simulink model "SomanetTuning"  (R2016b)
settings: Solver=FixedStepDiscrete  StartTime=0.0  StopTime=inf  FixedStep=0.002  RelTol=1e-3  EnableMultiTasking=on
libraries: slrtlib x14, dspstat3 x2, xpcethercatlib x1
(part 1 of 2)
settings Model: SimulationMode=external  Creator=march  LastModifiedBy=march
settings SolverCC: EnableConcurrentExecution=on  AutoInsertRateTranBlk=on
settings DataIOCC: SaveFormat=StructureWithTime
settings OptimizationCC: BlockReduction=off  OptimizeBlockIOStorage=off  BufferReuse=off  GlobalBufferReuse=off  ExpressionFolding=off  LocalBlockOutputs=off
settings HardwareCC: ProdBitPerPointer=32  ProdBitPerSizeT=32  ProdBitPerPtrDiffT=32  ProdLargestAtomicFloat=None  ProdWordSize=32  ProdLongLongMode=on  ProdHWDeviceType=Generic->32-bit x86 compatible
settings RTWCC: SystemTargetFile=slrt.tlc  TemplateMakefile=slrt_default_tmf  PostCodeGenCommand=SomanetTuning_make_rtw_hook  Description=Simulink Real-Time  RTWVerbose=off  CodeExecutionProfiling=on  RTWCompilerOptimization=on
settings SimulinkRealTimeCC: xPCModelTimeoutSecs=20

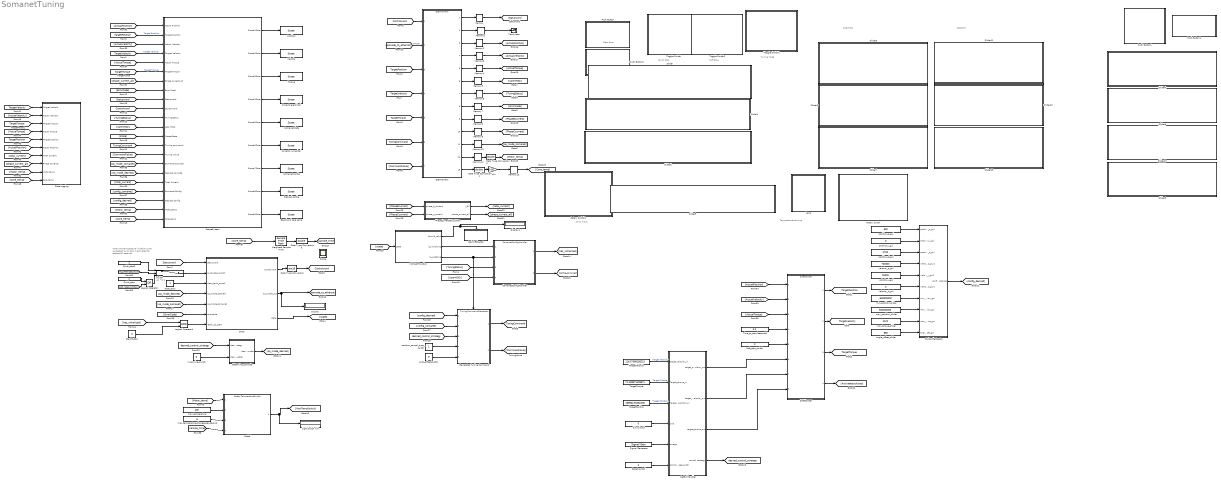
== system SomanetTuning ==
  note: VELOCITY
  note: POSITION
  note: Sinus Input
  note: Tuning Mode
  note: Quick Stop
  note: Clear Error
  note: When the temperature limitations are exceeded quick stop is activated for atleast 60 seconds
  note: Temperature-warning
  note: Soft Stop
  Board and core temp : slrtlib/Displays and Logging/Scope   scopeno=9  scopetype=Target  autostart=on  viewmode=Graphical rolling  formatstr='%15.6f'  grid=on  ylimits=[20,100]  nosamples=250  noprepostsamples=0  interleave=1  triggermode=FreeRun  triggersignal=1  trigsignalfromport=off  triggerlevel=0.0  triggerslope=Either  triggerscope=1  triggersample=0  filename=data.dat  mode=Lazy  writesize=512  autorestart=off  dynamicfilemode=off  maxwritefilesize=512*1024^2
  Chart : Stateflow chart  TreatAsAtomicUnit=on
  Currents graphical : slrtlib/Displays and Logging/Scope   scopeno=4  scopetype=Target  autostart=on  viewmode=Graphical sliding  formatstr='%15.6f'  grid=on  ylimits=[-30000,30000]  nosamples=500  noprepostsamples=0  interleave=1  triggermode=FreeRun  triggersignal=1  trigsignalfromport=off  triggerlevel=0.0  triggerslope=Either  triggerscope=1  triggersample=0  filename=data.dat  mode=Lazy  writesize=512  autorestart=off  dynamicfilemode=off  maxwritefilesize=512*1024^2
  Currents numerical : slrtlib/Displays and Logging/Scope   scopeno=6  scopetype=Target  autostart=on  viewmode=Numerical  formatstr='%15.6f'  grid=on  ylimits=[0,15000]  nosamples=500  noprepostsamples=0  interleave=1  triggermode=FreeRun  triggersignal=1  trigsignalfromport=off  triggerlevel=0.0  triggerslope=Either  triggerscope=1  triggersample=0  filename=data.dat  mode=Lazy  writesize=512  autorestart=off  dynamicfilemode=off  maxwritefilesize=512*1024^2
  Data Type Conversion : DataTypeConversion  OutDataTypeStr=uint16
  Data Type Conversion1 : DataTypeConversion  OutDataTypeStr=double
  Data Type Conversion2 : DataTypeConversion  OutDataTypeStr=double
  Data Type Conversion3 : DataTypeConversion  OutDataTypeStr=double
  Data logging : Subsystem
  Desired config : slrtlib/Displays and Logging/Scope   scopeno=8  scopetype=Target  autostart=on  viewmode=Numerical  formatstr='%15.0f'  grid=on  ylimits=[-600,600]  nosamples=500  noprepostsamples=0  interleave=1  triggermode=FreeRun  triggersignal=1  trigsignalfromport=off  triggerlevel=0.0  triggerslope=Either  triggerscope=1  triggersample=0  filename=data.dat  mode=Lazy  writesize=512  autorestart=off  dynamicfilemode=off  maxwritefilesize=512*1024^2
  Display : Display
  Display1 : Display
  EcatHandler : ModelReference  ModelNameDialog=EcatHandler  SimulationMode=Normal  ModelReferenceVersion=1.312
  Gain : Gain  Gain=0.05
  Generates Tuning Command : ModelReference  ModelNameDialog=TuningCommandGenerator.slx  SimulationMode=Normal  ModelReferenceVersion=1.298  EnablePortName=Enable  EnablePortStatesWhenEnabling=held
  GuiConfigCreator : Subsystem  TreatAsAtomicUnit=on
  Lamp : Subsystem  DialogController=hmiCreateDDGDialog  IsWebBlock=on  mask(MWDashboardBlock){webBlockId=994b938f-f4a1-444b-8998-3c3fe0212c8b, webBlockType=lamp, ShowInLibBrowser=on, ShowInitialText=on, HMISrcModelName=SomanetTuning}
      mask prompts: webBlockType "WebBlock Type"; HMISrcModelName "Source Model"
      mask help: SimulinkHMI:dialogs:LampDialogDesc
      mask Help: helpview([docroot '/mapfiles/simulink.map'], 'hmi_lamp')
      mask Display:
      | if strcmp(get_param(bdroot(gcb),'BlockDiagramType'), 'library')
      |     image([(matlabroot) '/toolbox/simulink/hmi/icons/Lamp.png']);
      | end
  Light Switch link : Display
  Logical Operator : Logic  Operator=OR  AllPortsSameDT=off  OutDataTypeStr=boolean
  Logical Operator1 : Logic  AllPortsSameDT=off  OutDataTypeStr=boolean
  MATLAB Function : MATLAB Function  TreatAsAtomicUnit=on
  Memory{,1..12} (13 alike) : Memory
  Model : ModelReference  ModelNameDialog=SafetyTemperatureSwitch.slx  SimulationMode=Normal  ModelReferenceVersion=1.310
  PhaseCurrentCalculation : Subsystem
  Position : slrtlib/Displays and Logging/Scope   scopeno=1  scopetype=Target  autostart=on  viewmode=Graphical sliding  formatstr='%15.6f'  grid=on  ylimits=[-5e6,5e6]  nosamples=500  noprepostsamples=0  interleave=1  triggermode=FreeRun  triggersignal=1  trigsignalfromport=off  triggerlevel=0.0  triggerslope=Either  triggerscope=1  triggersample=0  filename=data.dat  mode=Lazy  writesize=512  autorestart=off  dynamicfilemode=off  maxwritefilesize=512*1024^2
  Push Button : Subsystem  DialogController=hmiCreateDDGDialog  IsWebBlock=on  mask(MWDashboardBlock){webBlockId=356734de-af8c-46d0-90c2-8e8f664c98d9, webBlockType=pushbutton, ShowInLibBrwoser=on, ShowInitialText=on, HMISrcModelName=SomanetTuning}
      mask prompts: webBlockId "WebBlock Id"; webBlockType "WebBlock Type"; HMISrcModelName "Source Model"
      mask help: SimulinkHMI:dialogs:PushButtonDialogDesc
      mask Help: helpview([docroot '/mapfiles/simulink.map'], 'hmi_push_button')
      mask Display:
      | model = bdroot(gcb);
      | if strcmp(get_param(model,'BlockDiagramType'), 'library')
      |     image([(matlabroot) '/toolbox/simulink/hmi/icons/PushButton.png']);
      | end
  Push Button1 : Subsystem  DialogController=hmiCreateDDGDialog  IsWebBlock=on  mask(MWDashboardBlock){webBlockId=183612d4-71ac-4f8a-91dd-632476c1d2bb, webBlockType=pushbutton, ShowInLibBrwoser=on, ShowInitialText=on, HMISrcModelName=SomanetTuning}
      mask prompts: webBlockId "WebBlock Id"; webBlockType "WebBlock Type"; HMISrcModelName "Source Model"
      mask help: SimulinkHMI:dialogs:PushButtonDialogDesc
      mask Help: helpview([docroot '/mapfiles/simulink.map'], 'hmi_push_button')
      mask Display:
      | model = bdroot(gcb);
      | if strcmp(get_param(model,'BlockDiagramType'), 'library')
      |     image([(matlabroot) '/toolbox/simulink/hmi/icons/PushButton.png']);
      | end
  Push Button2 : Subsystem  DialogController=hmiCreateDDGDialog  IsWebBlock=on  mask(MWDashboardBlock){webBlockId=3a1387a3-9f18-4c83-b61d-eeb4a0f66ee7, webBlockType=pushbutton, ShowInLibBrwoser=on, ShowInitialText=on, HMISrcModelName=SomanetTuning}
      mask prompts: webBlockId "WebBlock Id"; webBlockType "WebBlock Type"; HMISrcModelName "Source Model"
      mask help: SimulinkHMI:dialogs:PushButtonDialogDesc
      mask Help: helpview([docroot '/mapfiles/simulink.map'], 'hmi_push_button')
      mask Display:
      | model = bdroot(gcb);
      | if strcmp(get_param(model,'BlockDiagramType'), 'library')
      |     image([(matlabroot) '/toolbox/simulink/hmi/icons/PushButton.png']);
      | end
  Push Button3 : Subsystem  DialogController=hmiCreateDDGDialog  IsWebBlock=on  mask(MWDashboardBlock){webBlockId=e281f3a8-d07c-4ea7-a33e-ce327e187917, webBlockType=pushbutton, ShowInLibBrwoser=on, ShowInitialText=on, HMISrcModelName=SomanetTuning}
      mask prompts: webBlockId "WebBlock Id"; webBlockType "WebBlock Type"; HMISrcModelName "Source Model"
      mask help: SimulinkHMI:dialogs:PushButtonDialogDesc
      mask Help: helpview([docroot '/mapfiles/simulink.map'], 'hmi_push_button')
      mask Display:
      | model = bdroot(gcb);
      | if strcmp(get_param(model,'BlockDiagramType'), 'library')
      |     image([(matlabroot) '/toolbox/simulink/hmi/icons/PushButton.png']);
      | end
  Quick_stop : Constant  OutDataTypeStr=boolean
  Quick_stop2 : Constant  OutDataTypeStr=boolean
  Reinit Ethercat : Subsystem
  Reset control : Constant  Value=0  OutDataTypeStr=int32
  Rotary Switch : Subsystem  DialogController=hmiCreateDDGDialog  IsWebBlock=on  mask(MWDashboardBlock){webBlockId=fa8f8082-b632-4cd3-875a-301596b55e06, webBlockType=discreteknob, ShowInLibBrowser=on, ShowInitialText=on, HMISrcModelName=SomanetTuning}
      mask prompts: webBlockId "WebBlock Id"; webBlockType "WebBlock Type"; HMISrcModelName "Source Model"
      mask help: SimulinkHMI:dialogs:DiscreteKnobDialogDesc
      mask Help: helpview([docroot '/mapfiles/simulink.map'], 'hmi_rotary_switch')
      mask Display:
      | model = bdroot(gcb);
      | if strcmp(get_param(model,'BlockDiagramType'), 'library')
      |     image([(matlabroot) '/toolbox/simulink/hmi/icons/DiscreteKnob.png']);
      | end
  Rotary Switch1 : Subsystem  DialogController=hmiCreateDDGDialog  IsWebBlock=on  mask(MWDashboardBlock){webBlockId=1d56b400-0412-44c3-8462-8cb9db8b7e4d, webBlockType=discreteknob, ShowInLibBrowser=on, ShowInitialText=on, HMISrcModelName=SomanetTuning}
      mask prompts: webBlockId "WebBlock Id"; webBlockType "WebBlock Type"; HMISrcModelName "Source Model"
      mask help: SimulinkHMI:dialogs:DiscreteKnobDialogDesc
      mask Help: helpview([docroot '/mapfiles/simulink.map'], 'hmi_rotary_switch')
      mask Display:
      | model = bdroot(gcb);
      | if strcmp(get_param(model,'BlockDiagramType'), 'library')
      |     image([(matlabroot) '/toolbox/simulink/hmi/icons/DiscreteKnob.png']);
      | end
  ScopeSystem : Subsystem
  SetGuiHandler : Subsystem
  Signal Generator : SignalGenerator  Frequency=0.281954887218
  "Sinus Input " : Constant  Value=0
  Slider : Subsystem  DialogController=hmiCreateDDGDialog  IsWebBlock=on  mask(MWDashboardBlock){webBlockId=d1263451-46af-4c55-8eeb-b2a1185fc98c, webBlockType=slider, ShowInLibBrowser=on, ShowInitialText=on, HMISrcModelName=SomanetTuning}
      mask prompts: webBlockId "WebBlock Id"; webBlockType "WebBlock Type"; HMISrcModelName "Source Model"
      mask help: SimulinkHMI:dialogs:SliderDialogDesc
      mask Help: helpview([docroot '/mapfiles/simulink.map'], 'hmi_slider')
      mask Display:
      | if strcmp(get_param(bdroot(gcb),'BlockDiagramType'), 'library')
      |     image([(matlabroot) '/toolbox/simulink/hmi/icons/Slider.png']);
      | end
  Slider1 : Subsystem  DialogController=hmiCreateDDGDialog  IsWebBlock=on  mask(MWDashboardBlock){webBlockId=e2636b5b-382c-42e0-acf3-b39c3266f57b, webBlockType=slider, ShowInLibBrowser=on, ShowInitialText=on, HMISrcModelName=SomanetTuning}
      mask prompts: webBlockId "WebBlock Id"; webBlockType "WebBlock Type"; HMISrcModelName "Source Model"
      mask help: SimulinkHMI:dialogs:SliderDialogDesc
      mask Help: helpview([docroot '/mapfiles/simulink.map'], 'hmi_slider')
      mask Display:
      | if strcmp(get_param(bdroot(gcb),'BlockDiagramType'), 'library')
      |     image([(matlabroot) '/toolbox/simulink/hmi/icons/Slider.png']);
      | end
  Slider10 : Subsystem  DialogController=hmiCreateDDGDialog  IsWebBlock=on  mask(MWDashboardBlock){webBlockId=def7d2a7-1287-4d64-81c3-00dc42338eac, webBlockType=slider, ShowInLibBrowser=on, ShowInitialText=on, HMISrcModelName=SomanetTuning}
      mask prompts: webBlockId "WebBlock Id"; webBlockType "WebBlock Type"; HMISrcModelName "Source Model"
      mask help: SimulinkHMI:dialogs:SliderDialogDesc
      mask Help: helpview([docroot '/mapfiles/simulink.map'], 'hmi_slider')
      mask Display:
      | if strcmp(get_param(bdroot(gcb),'BlockDiagramType'), 'library')
      |     image([(matlabroot) '/toolbox/simulink/hmi/icons/Slider.png']);
      | end
  Slider11 : Subsystem  DialogController=hmiCreateDDGDialog  IsWebBlock=on  mask(MWDashboardBlock){webBlockId=dc2b2cfc-71ae-4ea0-a0f2-7e0884df10cf, webBlockType=slider, ShowInLibBrowser=on, ShowInitialText=on, HMISrcModelName=SomanetTuning}
      mask prompts: webBlockId "WebBlock Id"; webBlockType "WebBlock Type"; HMISrcModelName "Source Model"
      mask help: SimulinkHMI:dialogs:SliderDialogDesc
      mask Help: helpview([docroot '/mapfiles/simulink.map'], 'hmi_slider')
      mask Display:
      | if strcmp(get_param(bdroot(gcb),'BlockDiagramType'), 'library')
      |     image([(matlabroot) '/toolbox/simulink/hmi/icons/Slider.png']);
      | end
  Slider12 : Subsystem  DialogController=hmiCreateDDGDialog  IsWebBlock=on  mask(MWDashboardBlock){webBlockId=7ae4c4dc-b42e-45e0-b891-75a3f1e5fd6f, webBlockType=slider, ShowInLibBrowser=on, ShowInitialText=on, HMISrcModelName=SomanetTuning}
      mask prompts: webBlockId "WebBlock Id"; webBlockType "WebBlock Type"; HMISrcModelName "Source Model"
      mask help: SimulinkHMI:dialogs:SliderDialogDesc
      mask Help: helpview([docroot '/mapfiles/simulink.map'], 'hmi_slider')
      mask Display:
      | if strcmp(get_param(bdroot(gcb),'BlockDiagramType'), 'library')
      |     image([(matlabroot) '/toolbox/simulink/hmi/icons/Slider.png']);
      | end
  Slider13 : Subsystem  DialogController=hmiCreateDDGDialog  IsWebBlock=on  mask(MWDashboardBlock){webBlockId=f6d04e87-2e98-45c4-b429-031f5ea3085d, webBlockType=slider, ShowInLibBrowser=on, ShowInitialText=on, HMISrcModelName=SomanetTuning}
      mask prompts: webBlockId "WebBlock Id"; webBlockType "WebBlock Type"; HMISrcModelName "Source Model"
      mask help: SimulinkHMI:dialogs:SliderDialogDesc
      mask Help: helpview([docroot '/mapfiles/simulink.map'], 'hmi_slider')
      mask Display:
      | if strcmp(get_param(bdroot(gcb),'BlockDiagramType'), 'library')
      |     image([(matlabroot) '/toolbox/simulink/hmi/icons/Slider.png']);
      | end
  Slider2 : Subsystem  DialogController=hmiCreateDDGDialog  IsWebBlock=on  mask(MWDashboardBlock){webBlockId=71234142-cef9-4b37-b6ab-ce5d7e36af05, webBlockType=slider, ShowInLibBrowser=on, ShowInitialText=on, HMISrcModelName=SomanetTuning}
      mask prompts: webBlockId "WebBlock Id"; webBlockType "WebBlock Type"; HMISrcModelName "Source Model"
      mask help: SimulinkHMI:dialogs:SliderDialogDesc
      mask Help: helpview([docroot '/mapfiles/simulink.map'], 'hmi_slider')
      mask Display:
      | if strcmp(get_param(bdroot(gcb),'BlockDiagramType'), 'library')
      |     image([(matlabroot) '/toolbox/simulink/hmi/icons/Slider.png']);
      | end
  Slider3 : Subsystem  DialogController=hmiCreateDDGDialog  IsWebBlock=on  mask(MWDashboardBlock){webBlockId=9cddd46d-1cb7-4126-ab3d-ebd7afdeb18b, webBlockType=slider, ShowInLibBrowser=on, ShowInitialText=on, HMISrcModelName=SomanetTuning}
      mask prompts: webBlockId "WebBlock Id"; webBlockType "WebBlock Type"; HMISrcModelName "Source Model"
      mask help: SimulinkHMI:dialogs:SliderDialogDesc
      mask Help: helpview([docroot '/mapfiles/simulink.map'], 'hmi_slider')
      mask Display:
      | if strcmp(get_param(bdroot(gcb),'BlockDiagramType'), 'library')
      |     image([(matlabroot) '/toolbox/simulink/hmi/icons/Slider.png']);
      | end
  Slider4 : Subsystem  DialogController=hmiCreateDDGDialog  IsWebBlock=on  mask(MWDashboardBlock){webBlockId=fa1a1418-0503-4b20-b29d-6741a8e61eb2, webBlockType=slider, ShowInLibBrowser=on, ShowInitialText=on, HMISrcModelName=SomanetTuning}
      mask prompts: webBlockId "WebBlock Id"; webBlockType "WebBlock Type"; HMISrcModelName "Source Model"
      mask help: SimulinkHMI:dialogs:SliderDialogDesc
      mask Help: helpview([docroot '/mapfiles/simulink.map'], 'hmi_slider')
      mask Display:
      | if strcmp(get_param(bdroot(gcb),'BlockDiagramType'), 'library')
      |     image([(matlabroot) '/toolbox/simulink/hmi/icons/Slider.png']);
      | end
  Slider5 : Subsystem  DialogController=hmiCreateDDGDialog  IsWebBlock=on  mask(MWDashboardBlock){webBlockId=e24694ff-6856-4d6d-8c39-63b50901b388, webBlockType=slider, ShowInLibBrowser=on, ShowInitialText=on, HMISrcModelName=SomanetTuning}
      mask prompts: webBlockId "WebBlock Id"; webBlockType "WebBlock Type"; HMISrcModelName "Source Model"
      mask help: SimulinkHMI:dialogs:SliderDialogDesc
      mask Help: helpview([docroot '/mapfiles/simulink.map'], 'hmi_slider')
      mask Display:
      | if strcmp(get_param(bdroot(gcb),'BlockDiagramType'), 'library')
      |     image([(matlabroot) '/toolbox/simulink/hmi/icons/Slider.png']);
      | end
  Slider6 : Subsystem  DialogController=hmiCreateDDGDialog  IsWebBlock=on  mask(MWDashboardBlock){webBlockId=8e804c44-8f02-4255-850c-29e295587076, webBlockType=slider, ShowInLibBrowser=on, ShowInitialText=on, HMISrcModelName=SomanetTuning}
      mask prompts: webBlockId "WebBlock Id"; webBlockType "WebBlock Type"; HMISrcModelName "Source Model"
      mask help: SimulinkHMI:dialogs:SliderDialogDesc
      mask Help: helpview([docroot '/mapfiles/simulink.map'], 'hmi_slider')
      mask Display:
      | if strcmp(get_param(bdroot(gcb),'BlockDiagramType'), 'library')
      |     image([(matlabroot) '/toolbox/simulink/hmi/icons/Slider.png']);
      | end
  Slider7 : Subsystem  DialogController=hmiCreateDDGDialog  IsWebBlock=on  mask(MWDashboardBlock){webBlockId=44154478-d107-4041-943a-7a09b0b07a14, webBlockType=slider, ShowInLibBrowser=on, ShowInitialText=on, HMISrcModelName=SomanetTuning}
      mask prompts: webBlockId "WebBlock Id"; webBlockType "WebBlock Type"; HMISrcModelName "Source Model"
      mask help: SimulinkHMI:dialogs:SliderDialogDesc
      mask Help: helpview([docroot '/mapfiles/simulink.map'], 'hmi_slider')
      mask Display:
      | if strcmp(get_param(bdroot(gcb),'BlockDiagramType'), 'library')
      |     image([(matlabroot) '/toolbox/simulink/hmi/icons/Slider.png']);
      | end
  Slider8 : Subsystem  DialogController=hmiCreateDDGDialog  IsWebBlock=on  mask(MWDashboardBlock){webBlockId=b2209b26-3c3d-4464-9b10-a7343f526e76, webBlockType=slider, ShowInLibBrowser=on, ShowInitialText=on, HMISrcModelName=SomanetTuning}
      mask prompts: webBlockId "WebBlock Id"; webBlockType "WebBlock Type"; HMISrcModelName "Source Model"
      mask help: SimulinkHMI:dialogs:SliderDialogDesc
      mask Help: helpview([docroot '/mapfiles/simulink.map'], 'hmi_slider')
      mask Display:
      | if strcmp(get_param(bdroot(gcb),'BlockDiagramType'), 'library')
      |     image([(matlabroot) '/toolbox/simulink/hmi/icons/Slider.png']);
      | end
  Slider9 : Subsystem  DialogController=hmiCreateDDGDialog  IsWebBlock=on  mask(MWDashboardBlock){webBlockId=4d3b8c13-4602-4919-8b6c-fd4a4d0fcea2, webBlockType=slider, ShowInLibBrowser=on, ShowInitialText=on, HMISrcModelName=SomanetTuning}
      mask prompts: webBlockId "WebBlock Id"; webBlockType "WebBlock Type"; HMISrcModelName "Source Model"
      mask help: SimulinkHMI:dialogs:SliderDialogDesc
      mask Help: helpview([docroot '/mapfiles/simulink.map'], 'hmi_slider')
      mask Display:
      | if strcmp(get_param(bdroot(gcb),'BlockDiagramType'), 'library')
      |     image([(matlabroot) '/toolbox/simulink/hmi/icons/Slider.png']);
      | end
  SoftStopper : ModelReference  ModelNameDialog=SoftStopper  SimulationMode=Normal  ModelReferenceVersion=1.307
  Soft_stop_switch : Constant  Value=0
  Somanet config : slrtlib/Displays and Logging/Scope   scopeno=7  scopetype=Target  autostart=on  viewmode=Numerical  formatstr='%15.0f'  grid=on  ylimits=[-600,600]  nosamples=500  noprepostsamples=0  interleave=1  triggermode=FreeRun  triggersignal=1  trigsignalfromport=off  triggerlevel=0.0  triggerslope=Either  triggerscope=1  triggersample=0  filename=data.dat  mode=Lazy  writesize=512  autorestart=off  dynamicfilemode=off  maxwritefilesize=512*1024^2
  Somanet data : slrtlib/Displays and Logging/Scope   scopeno=5  scopetype=Target  autostart=on  viewmode=Numerical  formatstr='%15.0f'  grid=on  ylimits=[-32000,32000]  nosamples=500  noprepostsamples=0  interleave=1  triggermode=FreeRun  triggersignal=1  trigsignalfromport=off  triggerlevel=0.0  triggerslope=Either  triggerscope=1  triggersample=0  filename=data.dat  mode=Lazy  writesize=512  autorestart=off  dynamicfilemode=off  maxwritefilesize=512*1024^2
  SomanetConfigHandler : ModelReference  ModelNameDialog=SomanetConfigHandler.slx  SimulationMode=Normal  ModelReferenceVersion=1.301
  Start Button : Constant  Value=0
  Switch : Switch  Criteria=u2 ~= 0  OutDataTypeStr=Inherit: Inherit via back propagation
  TargetPosition : Constant  Value=169902.91262136  OutDataTypeStr=double
  TargetTorque : Constant  Value=71.428571428571  OutDataTypeStr=double
  TargetVelocity : Constant  Value=116.57568238213  OutDataTypeStr=double
  Terminator : Terminator
  "Time_to_stop [seconds] " : Constant  Value=0.2
  Toggle Switch : Subsystem  DialogController=hmiCreateDDGDialog  IsWebBlock=on  mask(MWDashboardBlock){webBlockId=c1205c1e-d06e-42cd-b87b-d8f543a58887, webBlockType=toggleswitch, ShowInLibBrowser=on, ShowInitialText=on, HMISrcModelName=SomanetTuning}
      mask prompts: webBlockId "WebBlock Id"; webBlockType "WebBlock Type"; HMISrcModelName "Source Model"
      mask help: SimulinkHMI:dialogs:SwitchDialogDesc
      mask Help: helpview([docroot '/mapfiles/simulink.map'], 'hmi_toggle_switch')
      mask Display:
      | if strcmp(get_param(bdroot(gcb),'BlockDiagramType'), 'library')
      |     image([(matlabroot) '/toolbox/simulink/hmi/icons/ToggleSwitch.png']);
      | end
  Toggle Switch1 : Subsystem  DialogController=hmiCreateDDGDialog  IsWebBlock=on  mask(MWDashboardBlock){webBlockId=1668bd15-a3a5-45fe-adf4-1341c8503691, webBlockType=toggleswitch, ShowInLibBrowser=on, ShowInitialText=on, HMISrcModelName=SomanetTuning}
      mask prompts: webBlockId "WebBlock Id"; webBlockType "WebBlock Type"; HMISrcModelName "Source Model"
      mask help: SimulinkHMI:dialogs:SwitchDialogDesc
      mask Help: helpview([docroot '/mapfiles/simulink.map'], 'hmi_toggle_switch')
      mask Display:
      | if strcmp(get_param(bdroot(gcb),'BlockDiagramType'), 'library')
      |     image([(matlabroot) '/toolbox/simulink/hmi/icons/ToggleSwitch.png']);
      | end
  Toggle Switch2 : Subsystem  DialogController=hmiCreateDDGDialog  IsWebBlock=on  mask(MWDashboardBlock){webBlockId=8b935bd3-1501-4cdb-ad36-9f1bad2e5a66, webBlockType=toggleswitch, ShowInLibBrowser=on, ShowInitialText=on, HMISrcModelName=SomanetTuning}
      mask prompts: webBlockId "WebBlock Id"; webBlockType "WebBlock Type"; HMISrcModelName "Source Model"
      mask help: SimulinkHMI:dialogs:SwitchDialogDesc
      mask Help: helpview([docroot '/mapfiles/simulink.map'], 'hmi_toggle_switch')
      mask Display:
      | if strcmp(get_param(bdroot(gcb),'BlockDiagramType'), 'library')
      |     image([(matlabroot) '/toolbox/simulink/hmi/icons/ToggleSwitch.png']);
      | end
  Torque : slrtlib/Displays and Logging/Scope   scopeno=3  scopetype=Target  autostart=on  viewmode=Graphical sliding  formatstr='%15.6f'  grid=on  ylimits=[-600,600]  nosamples=250  noprepostsamples=0  interleave=1  triggermode=FreeRun  triggersignal=1  trigsignalfromport=off  triggerlevel=0.0  triggerslope=Either  triggerscope=1  triggersample=0  filename=data.dat  mode=Lazy  writesize=512  autorestart=off  dynamicfilemode=off  maxwritefilesize=512*1024^2
  Velocity : slrtlib/Displays and Logging/Scope   scopeno=2  scopetype=Target  autostart=on  viewmode=Graphical sliding  formatstr='%15.6f'  grid=on  ylimits=[-4000,4000]  nosamples=250  noprepostsamples=0  interleave=1  triggermode=FreeRun  triggersignal=1  trigsignalfromport=off  triggerlevel=0.0  triggerslope=Either  triggerscope=1  triggersample=0  filename=data.dat  mode=Lazy  writesize=512  autorestart=off  dynamicfilemode=off  maxwritefilesize=512*1024^2
  Weighted Sample Time : SampleTimeMath  TsampMathOp=Ts Only
  angle_offset_slider : Constant  Value=960  OutDataTypeStr=int32
  auto_offset_button : Constant  Value=0
  clear_error : Constant  OutDataTypeStr=boolean
  determine_opmode : Subsystem
  "livetuning_switch " : Constant  Value=0  OutDataTypeStr=boolean
  max_position_slider : Constant  Value=500000000  OutDataTypeStr=int32
  max_temperature : Constant  Value=100
  max_temperature_change_per_second : Constant  Value=5
  max_torque_slider : Constant  Value=2122  OutDataTypeStr=int32
  min_position_slider : Constant  Value=-500000000  OutDataTypeStr=int32
  position_control_type_switch : Constant  OutDataTypeStr=int32
  position_d_gui : Constant  Value=2700  OutDataTypeStr=int32
  position_i_gui : Constant  Value=0  OutDataTypeStr=int32
  position_p_gui : Constant  Value=600  OutDataTypeStr=int32
  velocity_d_gui : Constant  Value=0  OutDataTypeStr=int32
  velocity_i_gui : Constant  Value=20000  OutDataTypeStr=int32
  velocity_p_gui : Constant  Value=700000  OutDataTypeStr=int32
  Scope : Scope
  tag scope: Controlword=global, Statusword=global, TargetPosition=global, TargetTorque=global, TargetVelocity=global, TuningCommand=global, desired_control_strategy=global
  wires:
  Chart/1(controlword) -> Data Type Conversion/1
  Switch/1 -> Chart/2(quick_stop_switch)
  clear_error/1 -> Chart/3(clear_fault_switch)
  Data Type Conversion/1 -> [Controlword]
  [Statusword] -> Chart/1(statusword)
  Chart/2(op_mode_out) -> [opmode_to_ethercat], Display/1
  [op_mode_somanet] -> Chart/5(op_mode_somanet)
  [op_mode_desired] -> Chart/4(op_mode_desired)
  Chart/3(state) -> [state]
  determine_opmode/1(desired_opmode) -> [op_mode_desired]
  velocity_p_gui/1 -> GuiConfigCreator/4(velocity_p_gui1)
  velocity_i_gui/1 -> GuiConfigCreator/5(velocity_i_gui1)
  velocity_d_gui/1 -> GuiConfigCreator/6(velocity_d_gui1)
  min_position_slider/1 -> GuiConfigCreator/7(min_position_gui)
  angle_offset_slider/1 -> GuiConfigCreator/10(angle_offset_gui)
  position_i_gui/1 -> GuiConfigCreator/2(position_i_gui)
  max_position_slider/1 -> GuiConfigCreator/8(max_position_gui)
  max_torque_slider/1 -> GuiConfigCreator/9(max_torque_gui)
  position_d_gui/1 -> GuiConfigCreator/3(position_d_gui)
  position_p_gui/1 -> GuiConfigCreator/1(position_p_gui)
  GuiConfigCreator/1(config_desired) -> [config_desired]
  [desired_control_strategy] -> determine_opmode/1(desired_control_strategy)
  "livetuning_switch "/1 -> determine_opmode/2(desired_somanet_state)
  [state] -> MATLAB Function/1(state)
  MATLAB Function/2(is_initializing) -> SomanetConfigHandler/1
  MATLAB Function/3(is_updating) -> Generates Tuning Command/Enable, SomanetConfigHandler/2
  [UserMISO] -> SomanetConfigHandler/4
  [TuningStatus] -> SomanetConfigHandler/3
  SomanetConfigHandler/1 -> [has_initialized]
  SomanetConfigHandler/2 -> [config_somanet]
  position_control_type_switch/1 -> Generates Tuning Command/4
  [desired_control_strategy] -> Generates Tuning Command/3
  [config_desired] -> Generates Tuning Command/1
  [config_somanet] -> Generates Tuning Command/2
  auto_offset_button/1 -> Generates Tuning Command/5
  [PhaseBcurrent] -> PhaseCurrentCalculation/1(phase_b_current)
  [PhaseCcurrent] -> PhaseCurrentCalculation/2(phase_c_current)
  PhaseCurrentCalculation/1(I_DC) -> [total_current]
  PhaseCurrentCalculation/2(phase_current_all) -> [phase_current_all]
  ScopeSystem/2(Scope2Data) -> Velocity/1
  ScopeSystem/1(Scope1Data) -> Position/1
  ScopeSystem/3(Scope3Data) -> Torque/1
  ScopeSystem/4(Scope4Data) -> Currents graphical/1
  ScopeSystem/5(Scope5Data) -> Somanet data/1
  ScopeSystem/6(Scope6Data) -> Currents numerical/1
  ScopeSystem/7(Scope7Data) -> Somanet config/1
  [ActualVelocity] -> ScopeSystem/3(Actual Velocity)
  [ActualTorque] -> ScopeSystem/5(Actual Torque)
  [ActualPosition] -> ScopeSystem/1(Actual Position)
  [phase_current_all] -> ScopeSystem/7(Phase currents all)
  [TargetPosition] -> ScopeSystem/2(Target Position)  "Target Position"
  [TuningStatus] -> ScopeSystem/11("Tuningstatus ")
  [UserMISO] -> ScopeSystem/12("User MISO ")
  [config_somanet] -> ScopeSystem/19(Somanet Config)
  [config_desired] -> ScopeSystem/20(Desired Config)
  [total_current] -> ScopeSystem/18(Total Current)
  [TargetVelocity] -> ScopeSystem/4(Target Velocity)  "Target Velocity"
  [ErrorCode] -> ScopeSystem/8(Error Code)
  [op_mode_somanet] -> ScopeSystem/16(Somanet opmode)
  [op_mode_desired] -> ScopeSystem/17(Desired opmode)
  [Controlword] -> ScopeSystem/10(Controlword)
  [TuningCommand] -> ScopeSystem/14(Tuning command)
  [CommandValue] -> ScopeSystem/15(Tuning value)
  [TargetTorque] -> ScopeSystem/6(Target Torque)  "Target Torque"
  [Statusword] -> ScopeSystem/9(Statusword)
  [state] -> ScopeSystem/13(MasterState)
  Generates Tuning Command/2 -> [CommandValue]
  Generates Tuning Command/1 -> [TuningCommand]
  ScopeSystem/8(Scope8Data) -> Desired config/1
  [ErrorCode] -> Chart/6(errorcode)
  MATLAB Function/1(should_reinit) -> Reinit Ethercat/Enable, Display1/1
  [ActualTorque] -> Data logging/4(Actual Torque)
  [TargetVelocity] -> Data logging/1(Target Velocity)
  [ActualVelocity] -> Data logging/2(Actual Velocity)
  [TargetTorque] -> Data logging/3(Target Torque)
  [TargetPosition] -> Data logging/5(Target position)
  [ActualPosition] -> Data logging/6(Actual Position)
  [total_current] -> Data logging/7(Total Current)
  [phase_current_all] -> Data logging/8(Phase Currents)
  [Motor_temp] -> Model/1
  Model/1 -> Light Switch link/1, [MaxTempSwitch]
  max_temperature/1 -> Model/2
  max_temperature_change_per_second/1 -> Model/3
  Quick_stop2/1 -> Switch/1
  [Motor_temp] -> ScopeSystem/21(Motor_temp)
  [Core_temp] -> ScopeSystem/22(Core_temp)
  [Core_temp] -> Data logging/10(Core temp)
  [Motor_temp] -> Data logging/9(Motor temp)
  Data Type Conversion1/1 -> Gain/1
  Gain/1 -> Memory12/1
  [ActualPosition] -> SoftStopper/1
  [ActualVelocity] -> SoftStopper/2
  [ActualTorque] -> SoftStopper/3
  "Time_to_stop [seconds] "/1 -> SoftStopper/4
  Soft_stop_switch/1 -> SoftStopper/5
  TargetVelocity/1 -> SetGuiHandler/1(target_velocity_in)  "Target Velocity"
  TargetTorque/1 -> SetGuiHandler/2(Target_torque_in)  "Target Torque"
  TargetPosition/1 -> SetGuiHandler/3(Target_position_in)  "Target Position"
  "Sinus Input "/1 -> SetGuiHandler/4(sine)
  Signal Generator/1 -> SetGuiHandler/5(omega)
  Reset control/1 -> SetGuiHandler/6(control_reset_switch)
  [MaxTempSwitch] -> Switch/2
  Quick_stop/1 -> Logical Operator/1
  [Activatequickstop] -> Logical Operator/2
  Logical Operator/1 -> Switch/3
  ScopeSystem/9(Scope9Data) -> Board and core temp/1
  SoftStopper/1 -> [TargetPosition]
  SoftStopper/2 -> [TargetVelocity]
  SoftStopper/3 -> [TargetTorque]
  SoftStopper/4 -> [Activatequickstop]
  SetGuiHandler/4(control strategy) -> [desired_control_strategy]
  SetGuiHandler/1(target_position_out) -> SoftStopper/6
  SetGuiHandler/2(target_velocity_out) -> SoftStopper/7
  SetGuiHandler/3(target_torque_out) -> SoftStopper/8
  [Controlword] -> EcatHandler/1
  [opmode_to_ethercat] -> EcatHandler/2  "pMode"
  [TargetPosition] -> EcatHandler/3
  [TargetVelocity] -> EcatHandler/4
  [TargetTorque] -> EcatHandler/5
  [TuningCommand] -> EcatHandler/6
  [CommandValue] -> EcatHandler/7
  EcatHandler/1 -> Memory/1
  EcatHandler/2 -> Memory1/1
  EcatHandler/3 -> Memory2/1
  EcatHandler/4 -> Memory3/1
  EcatHandler/5 -> Memory4/1
  EcatHandler/6 -> Memory5/1
  EcatHandler/7 -> Memory6/1
  EcatHandler/8 -> Memory7/1
  EcatHandler/9 -> Memory8/1
  EcatHandler/10 -> Memory9/1
  EcatHandler/11 -> Memory10/1
  EcatHandler/12 -> Memory11/1
  Memory/1 -> [Statusword]
  Memory1/1 -> Terminator/1
  Memory2/1 -> [ActualPosition]
  Memory3/1 -> [ActualVelocity]
  Memory4/1 -> [ActualTorque]
  Memory5/1 -> [UserMISO]
  Memory6/1 -> [TuningStatus]
  Memory7/1 -> [ErrorCode]
  Memory8/1 -> [PhaseBcurrent]
  Memory9/1 -> [PhaseCcurrent]
  Memory10/1 -> [op_mode_somanet]
  Memory11/1 -> Data Type Conversion2/1
  EcatHandler/13 -> Data Type Conversion1/1
  Memory12/1 -> [Core_temp]
  Logical Operator1/1 -> Chart/7(ready_to_start)
  [has_initialized] -> Logical Operator1/1
  Start Button/1 -> Logical Operator1/2
  [sample_time] -> Model/4
  Data Type Conversion3/1 -> [sample_time]
  Weighted Sample Time/1 -> Data Type Conversion3/1
  [Core_temp] -> Weighted Sample Time/1
  Data Type Conversion2/1 -> [Motor_temp]

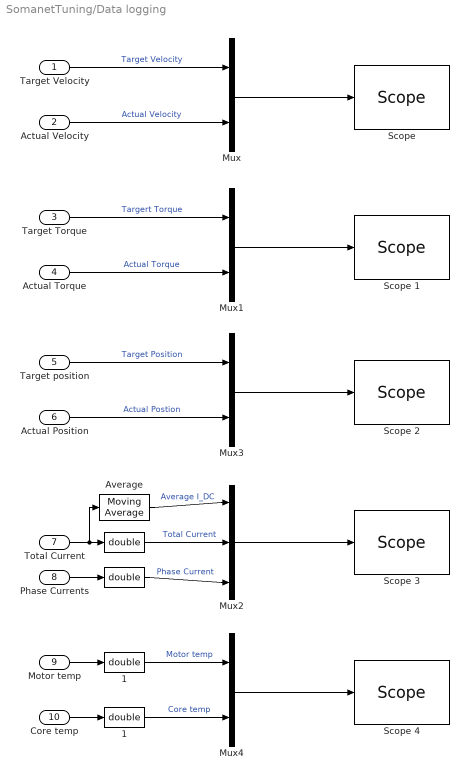
== system SomanetTuning/Data logging ==
  Target Velocity : Inport
  Actual Velocity : Inport  Port=2
  Target Torque : Inport  Port=3
  Actual Torque : Inport  Port=4
  Target position : Inport  Port=5
  Actual Position : Inport  Port=6
  Total Current : Inport  Port=7
  Phase Currents : Inport  Port=8
  Motor temp : Inport  Port=9
  Core temp : Inport  Port=10
   {,,1,1} (4 alike) : DataTypeConversion  OutDataTypeStr=double
  " Average" : dspstat3/Moving Average  Method=Sliding window  SpecifyWindowLength=on  WindowLength=10  ForgettingFactor=0.9  SimulateUsing=Code generation
  Mux{,1,3..4} (4 alike) : Mux  Inputs=2
  Mux2 : Mux  Inputs=3
  "Scope " : slrtlib/Displays and Logging/Scope   scopeno=10  scopetype=File  autostart=on  viewmode=Graphical redraw  formatstr='%15.6f'  grid=on  ylimits=[0,0]  nosamples=1000000  noprepostsamples=0  interleave=1  triggermode=FreeRun  triggersignal=1  trigsignalfromport=off  triggerlevel=0.0  triggerslope=Either  triggerscope=1  triggersample=0  filename=velocity.dat  mode=Lazy  writesize=512  autorestart=off  dynamicfilemode=off  maxwritefilesize=512*1024^2
  Scope 1 : slrtlib/Displays and Logging/Scope   scopeno=11  scopetype=File  autostart=on  viewmode=Graphical redraw  formatstr='%15.6f'  grid=on  ylimits=[0,0]  nosamples=1000000  noprepostsamples=0  interleave=1  triggermode=FreeRun  triggersignal=1  trigsignalfromport=off  triggerlevel=0.0  triggerslope=Either  triggerscope=1  triggersample=0  filename=torque.dat  mode=Lazy  writesize=512  autorestart=off  dynamicfilemode=off  maxwritefilesize=512*1024^2
  Scope 2 : slrtlib/Displays and Logging/Scope   scopeno=12  scopetype=File  autostart=on  viewmode=Graphical redraw  formatstr='%15.6f'  grid=on  ylimits=[0,0]  nosamples=1000000  noprepostsamples=0  interleave=1  triggermode=FreeRun  triggersignal=1  trigsignalfromport=off  triggerlevel=0.0  triggerslope=Either  triggerscope=1  triggersample=0  filename=position.dat  mode=Lazy  writesize=512  autorestart=off  dynamicfilemode=off  maxwritefilesize=512*1024^2
  Scope 3 : slrtlib/Displays and Logging/Scope   scopeno=13  scopetype=File  autostart=on  viewmode=Graphical redraw  formatstr='%15.6f'  grid=on  ylimits=[0,0]  nosamples=1000000  noprepostsamples=0  interleave=1  triggermode=FreeRun  triggersignal=1  trigsignalfromport=off  triggerlevel=0.0  triggerslope=Either  triggerscope=1  triggersample=0  filename=current.dat  mode=Lazy  writesize=512  autorestart=off  dynamicfilemode=off  maxwritefilesize=512*1024^2
  Scope 4 : slrtlib/Displays and Logging/Scope   scopeno=14  scopetype=File  autostart=on  viewmode=Graphical redraw  formatstr='%15.6f'  grid=on  ylimits=[0,0]  nosamples=1000000  noprepostsamples=0  interleave=1  triggermode=FreeRun  triggersignal=1  trigsignalfromport=off  triggerlevel=0.0  triggerslope=Either  triggerscope=1  triggersample=0  filename=temp.dat  mode=Lazy  writesize=512  autorestart=off  dynamicfilemode=off  maxwritefilesize=512*1024^2
  wires:
  Target Velocity/1 -> Mux/1  "Target Velocity"
  Actual Velocity/1 -> Mux/2  "Actual Velocity"
  Total Current/1 -> " Average"/1, " "/1
  Phase Currents/1 -> " "/1
  Actual Position/1 -> Mux3/2  "Actual Postion"
  Target position/1 -> Mux3/1  "Target Position"
  Actual Torque/1 -> Mux1/2  "Actual Torque"
  Target Torque/1 -> Mux1/1  "Targert Torque"
  Mux2/1 -> Scope 3/1
  Mux3/1 -> Scope 2/1
  Mux1/1 -> Scope 1/1
  Mux/1 -> "Scope "/1
  " "/1 -> Mux2/2  "Total Current"
  " "/1 -> Mux2/3  "Phase Current"
  Motor temp/1 -> " 1"/1
  Core temp/1 -> " 1"/1
  Mux4/1 -> Scope 4/1
  " 1"/1 -> Mux4/1  "Motor temp"
  " 1"/1 -> Mux4/2  "Core temp"
  " Average"/1 -> Mux2/1  "Average I_DC"

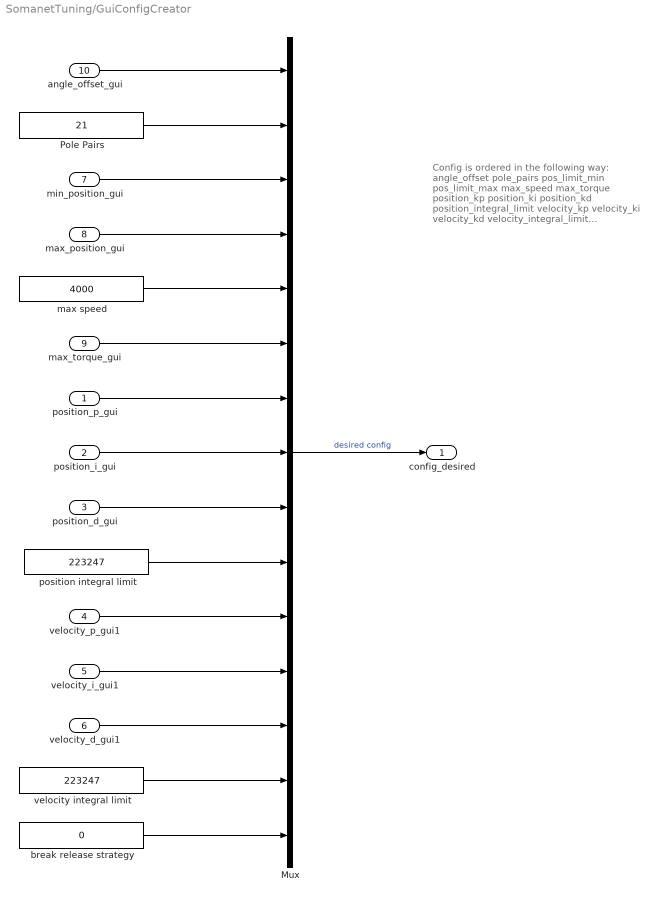
== system SomanetTuning/GuiConfigCreator ==
  note: Config is ordered in the following way:
      | angle_offset
      | pole_pairs
      | pos_limit_min
      | pos_limit_max
      | max_speed
      | max_torque
      | position_kp
      | position_ki
      | position_kd
      | position_integral_limit
      | velocity_kp
      | velocity_ki
      | velocity_kd
      | velocity_integral_limit
      | break_release_strategy
  position_p_gui : Inport  OutDataTypeStr=int32
  position_i_gui : Inport  Port=2  OutDataTypeStr=int32
  position_d_gui : Inport  Port=3  OutDataTypeStr=int32
  velocity_p_gui1 : Inport  Port=4  OutDataTypeStr=int32
  velocity_i_gui1 : Inport  Port=5  OutDataTypeStr=int32
  velocity_d_gui1 : Inport  Port=6  OutDataTypeStr=int32
  min_position_gui : Inport  Port=7  OutDataTypeStr=int32
  max_position_gui : Inport  Port=8  OutDataTypeStr=int32
  max_torque_gui : Inport  Port=9  OutDataTypeStr=int32
  angle_offset_gui : Inport  Port=10  OutDataTypeStr=int32
  Mux : Mux  Inputs=15
  Pole Pairs : Constant  Value=21  OutMin=[0]  OutDataTypeStr=int32
  "break release strategy " : Constant  Value=0  OutDataTypeStr=int32
  max speed : Constant  Value=4000  OutDataTypeStr=int32
  position integral limit : Constant  Value=223247  OutDataTypeStr=int32
  velocity integral limit : Constant  Value=223247  OutDataTypeStr=int32
  config_desired : Outport
  wires:
  max speed/1 -> Mux/5
  Pole Pairs/1 -> Mux/2
  position integral limit/1 -> Mux/10
  "break release strategy "/1 -> Mux/15
  min_position_gui/1 -> Mux/3
  angle_offset_gui/1 -> Mux/1
  max_position_gui/1 -> Mux/4
  velocity integral limit/1 -> Mux/14
  Mux/1 -> config_desired/1  "desired config"
  max_torque_gui/1 -> Mux/6
  position_p_gui/1 -> Mux/7
  position_i_gui/1 -> Mux/8
  position_d_gui/1 -> Mux/9
  velocity_p_gui1/1 -> Mux/11
  velocity_i_gui1/1 -> Mux/12
  velocity_d_gui1/1 -> Mux/13

== system SomanetTuning/Lamp ==

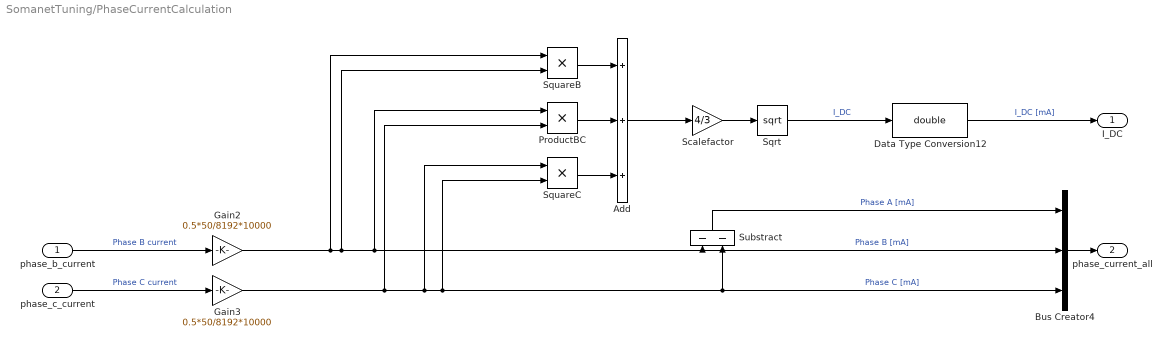
== system SomanetTuning/PhaseCurrentCalculation ==
  phase_b_current : Inport
  phase_c_current : Inport  Port=2
  Add : Sum  Inputs=+++
  Bus Creator4 : BusCreator  Inputs=3
  Data Type Conversion12 : DataTypeConversion  OutDataTypeStr=double
  Gain2 : Gain  Gain=0.5*50/8192*10000  OutDataTypeStr=double
  Gain3 : Gain  Gain=0.5*50/8192*10000  OutDataTypeStr=double
  ProductBC : Product  Inputs=**
  Scalefactor : Gain  Gain=4/3
  Sqrt : Sqrt  SaturateOnIntegerOverflow=on
  SquareB : Product  Inputs=**
  SquareC : Product  Inputs=**
  Substract : Sum  Inputs=--  OutDataTypeStr=double
  I_DC : Outport
  phase_current_all : Outport  Port=2
  wires:
  Bus Creator4/1 -> phase_current_all/1
  phase_b_current/1 -> Gain2/1  "Phase B current"
  Data Type Conversion12/1 -> I_DC/1  "I_DC [mA]"
  Substract/1 -> Bus Creator4/1  "Phase A [mA]"
  Gain2/1 -> SquareB/1, SquareB/2, ProductBC/1, Bus Creator4/2, Substract/1  "Phase B [mA]"
  phase_c_current/1 -> Gain3/1  "Phase C current"
  Sqrt/1 -> Data Type Conversion12/1  "I_DC"
  Gain3/1 -> ProductBC/2, SquareC/1, SquareC/2, Bus Creator4/3, Substract/2  "Phase C [mA]"
  SquareB/1 -> Add/1
  ProductBC/1 -> Add/2
  SquareC/1 -> Add/3
  Add/1 -> Scalefactor/1
  Scalefactor/1 -> Sqrt/1

== system SomanetTuning/Push Button ==

== system SomanetTuning/Push Button1 ==

== system SomanetTuning/Push Button2 ==

== system SomanetTuning/Push Button3 ==

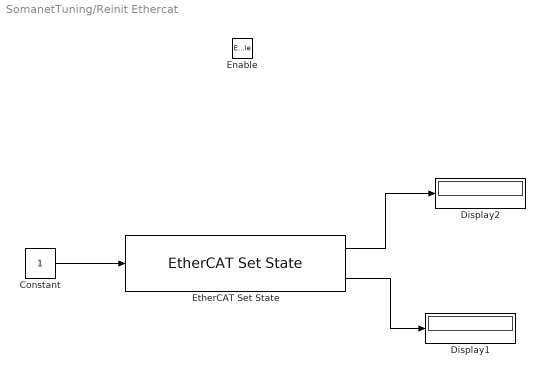
== system SomanetTuning/Reinit Ethercat ==
  Enable : EnablePort
  Constant : Constant  OutDataTypeStr=int32
  Display1 : Display
  Display2 : Display
  "EtherCAT Set State " : xpcethercatlib/EtherCAT Set State   device_id=0  timeout=0  sample_time=0
  wires:
  Constant/1 -> "EtherCAT Set State "/1
  "EtherCAT Set State "/1 -> Display2/1
  "EtherCAT Set State "/2 -> Display1/1

== system SomanetTuning/Rotary Switch ==

== system SomanetTuning/Rotary Switch1 ==

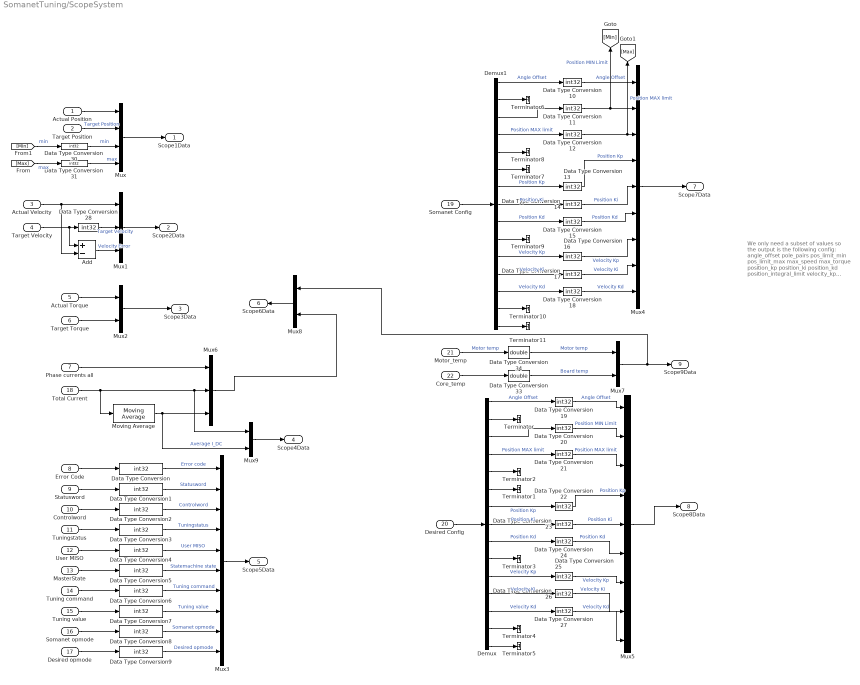
== system SomanetTuning/ScopeSystem ==
  note: We only need a subset of values
      | so the output is the following config:
      | angle_offset
      | pole_pairs
      | pos_limit_min
      | pos_limit_max
      | max_speed
      | max_torque
      | position_kp
      | position_ki
      | position_kd
      | position_integral_limit
      | velocity_kp
      | velocity_ki
      | velocity_kd
      | velocity_integral_limit
      | break_release_strategy
  Actual Position : Inport
  Target Position : Inport  Port=2
  Actual Velocity : Inport  Port=3
  Target Velocity : Inport  Port=4
  Actual Torque : Inport  Port=5
  Target Torque : Inport  Port=6
  Phase currents all : Inport  Port=7
  Error Code : Inport  Port=8
  Statusword : Inport  Port=9
  Controlword : Inport  Port=10
  "Tuningstatus " : Inport  Port=11
  "User MISO " : Inport  Port=12
  MasterState : Inport  Port=13
  Tuning command : Inport  Port=14
  Tuning value : Inport  Port=15
  Somanet opmode : Inport  Port=16
  Desired opmode : Inport  Port=17
  Total Current : Inport  Port=18
  Somanet Config : Inport  Port=19
  Desired Config : Inport  Port=20
  Motor_temp : Inport  Port=21
  Core_temp : Inport  Port=22
  Add : Sum  Inputs=+-
  Data Type Conversion{,1..28,30..31} (31 alike) : DataTypeConversion  OutDataTypeStr=int32
  Data Type Conversion33 : DataTypeConversion  OutDataTypeStr=double
  Data Type Conversion34 : DataTypeConversion  OutDataTypeStr=double
  Demux : Demux  Outputs=15
  Demux1 : Demux  Outputs=15
  Moving Average : dspstat3/Moving Average  Method=Sliding window  SpecifyWindowLength=on  WindowLength=10  ForgettingFactor=0.9  SimulateUsing=Code generation
  Mux : Mux
  Mux1 : Mux  Inputs=3
  Mux{2,7..9} (4 alike) : Mux  Inputs=2
  Mux3 : Mux  Inputs=10
  Mux4 : Mux  Inputs=9
  Mux5 : Mux  Inputs=9
  Mux6 : Mux  Inputs=3
  Terminator{,1..11} (12 alike) : Terminator
  Scope1Data : Outport
  Scope2Data : Outport  Port=2
  Scope3Data : Outport  Port=3
  Scope4Data : Outport  Port=4
  Scope5Data : Outport  Port=5
  Scope6Data : Outport  Port=6
  Scope7Data : Outport  Port=7
  Scope8Data : Outport  Port=8
  Scope9Data : Outport  Port=9
  wires:
  Target Position/1 -> Mux/2  "Target Position"
  Actual Position/1 -> Mux/1
  Mux/1 -> Scope1Data/1
  Target Velocity/1 -> Data Type Conversion28/1, Add/1
  Actual Velocity/1 -> Mux1/1, Add/2
  Mux1/1 -> Scope2Data/1
  Target Torque/1 -> Mux2/2
  Actual Torque/1 -> Mux2/1
  Mux2/1 -> Scope3Data/1
  "User MISO "/1 -> Data Type Conversion4/1
  "Tuningstatus "/1 -> Data Type Conversion3/1
  Error Code/1 -> Data Type Conversion/1
  Statusword/1 -> Data Type Conversion1/1
  MasterState/1 -> Data Type Conversion5/1
  Tuning command/1 -> Data Type Conversion6/1
  Tuning value/1 -> Data Type Conversion7/1
  Desired opmode/1 -> Data Type Conversion9/1
  Somanet opmode/1 -> Data Type Conversion8/1
  Controlword/1 -> Data Type Conversion2/1
  Mux3/1 -> Scope5Data/1
  Data Type Conversion/1 -> Mux3/1  "Error code"
  Data Type Conversion1/1 -> Mux3/2  "Statusword"
  Data Type Conversion2/1 -> Mux3/3  "Controlword"
  Data Type Conversion3/1 -> Mux3/4  "Tuningstatus"
  Data Type Conversion4/1 -> Mux3/5  "User MISO"
  Data Type Conversion5/1 -> Mux3/6  "Statemachine state"
  Data Type Conversion6/1 -> Mux3/7  "Tuning command"
  Data Type Conversion7/1 -> Mux3/8  "Tuning value"
  Data Type Conversion8/1 -> Mux3/9  "Somanet opmode"
  Data Type Conversion9/1 -> Mux3/10  "Desired opmode"
  Desired Config/1 -> Demux/1
  Demux/1 -> Data Type Conversion19/1  "Angle Offset"
  Demux/2 -> Terminator/1
  Demux/3 -> Data Type Conversion20/1
  Demux/4 -> Data Type Conversion21/1  "Position MAX limit"
  Demux/5 -> Terminator2/1
  Demux/6 -> Terminator1/1
  Demux/7 -> Data Type Conversion22/1  "Position Kp"
  Demux/8 -> Data Type Conversion23/1  "Position Ki"
  Demux/9 -> Data Type Conversion24/1  "Position Kd"
  Demux/10 -> Terminator3/1
  Demux/11 -> Data Type Conversion25/1  "Velocity Kp"
  Demux/12 -> Data Type Conversion26/1  "Velocity Ki"
  Demux/13 -> Data Type Conversion27/1  "Velocity Kd"
  Demux/14 -> Terminator4/1
  Demux/15 -> Terminator5/1
  Mux5/1 -> Scope8Data/1
  Data Type Conversion19/1 -> Mux5/1  "Angle Offset"
  Data Type Conversion20/1 -> Mux5/2  "Position MIN Limit"
  Data Type Conversion21/1 -> Mux5/3  "Position MAX limit"
  Data Type Conversion22/1 -> Mux5/4  "Position Kp"
  Data Type Conversion23/1 -> Mux5/5  "Position Ki"
  Data Type Conversion24/1 -> Mux5/6  "Position Kd"
  Data Type Conversion25/1 -> Mux5/7  "Velocity Kp"
  Data Type Conversion26/1 -> Mux5/8  "Velocity Ki"
  Data Type Conversion27/1 -> Mux5/9  "Velocity Kd"
  Demux1/1 -> Data Type Conversion10/1  "Angle Offset"
  Demux1/2 -> Terminator6/1
  Demux1/3 -> Data Type Conversion11/1
  Demux1/4 -> Data Type Conversion12/1  "Position MAX limit"
  Demux1/5 -> Terminator8/1
  Demux1/6 -> Terminator7/1
  Demux1/7 -> Data Type Conversion13/1  "Position Kp"
  Demux1/8 -> Data Type Conversion14/1  "Position Ki"
  Demux1/9 -> Data Type Conversion15/1  "Position Kd"
  Demux1/10 -> Terminator9/1
  Demux1/11 -> Data Type Conversion16/1  "Velocity Kp"
  Demux1/12 -> Data Type Conversion17/1  "Velocity Ki"
  Demux1/13 -> Data Type Conversion18/1  "Velocity Kd"
  Demux1/14 -> Terminator10/1
  Demux1/15 -> Terminator11/1
  Mux4/1 -> Scope7Data/1
  Data Type Conversion10/1 -> Mux4/1  "Angle Offset"
  Data Type Conversion11/1 -> Mux4/2, [Min]  "Position MIN Limit"
  Data Type Conversion12/1 -> [Max], Mux4/3  "Position MAX limit"
  Data Type Conversion13/1 -> Mux4/4  "Position Kp"
  Data Type Conversion14/1 -> Mux4/5  "Position Ki"
  Data Type Conversion15/1 -> Mux4/6  "Position Kd"
  Data Type Conversion16/1 -> Mux4/7  "Velocity Kp"
  Data Type Conversion17/1 -> Mux4/8  "Velocity Ki"
  Data Type Conversion18/1 -> Mux4/9  "Velocity Kd"
  Somanet Config/1 -> Demux1/1
  [Max] -> Data Type Conversion31/1  "max"
  [Min] -> Data Type Conversion30/1  "min"
  Phase currents all/1 -> Mux6/1
  Total Current/1 -> Moving Average/1, Mux9/1, Mux6/2
  Data Type Conversion30/1 -> Mux/3  "min"
  Data Type Conversion31/1 -> Mux/4  "max"
  Core_temp/1 -> Data Type Conversion33/1
  Motor_temp/1 -> Data Type Conversion34/1  "Motor temp"
  Data Type Conversion33/1 -> Mux7/2  "Board temp"
  Mux7/1 -> Mux8/1, Scope9Data/1
  Data Type Conversion34/1 -> Mux7/1  "Motor temp"
  Mux8/1 -> Scope6Data/1
  Mux6/1 -> Mux8/2
  Moving Average/1 -> Mux6/3, Mux9/2  "Average I_DC"
  Mux9/1 -> Scope4Data/1
  Add/1 -> Mux1/3  "Velocity Error"
  Data Type Conversion28/1 -> Mux1/2  "Target Velocity"

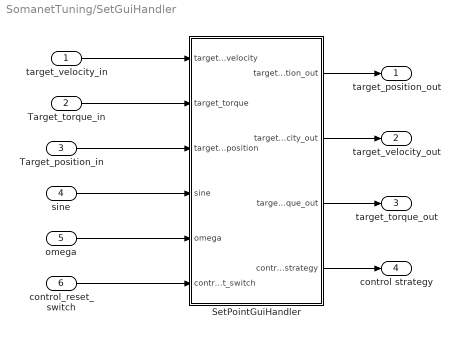
== system SomanetTuning/SetGuiHandler ==
  target_velocity_in : Inport
  Target_torque_in : Inport  Port=2
  Target_position_in : Inport  Port=3
  sine : Inport  Port=4
  omega : Inport  Port=5
  control_reset_switch : Inport  Port=6
  SetPointGuiHandler : Subsystem
  target_position_out : Outport
  target_velocity_out : Outport  Port=2
  target_torque_out : Outport  Port=3
  control strategy : Outport  Port=4
  wires:
  target_velocity_in/1 -> SetPointGuiHandler/1("target_velocity ")
  Target_position_in/1 -> SetPointGuiHandler/3(target_position)
  sine/1 -> SetPointGuiHandler/4(sine)
  Target_torque_in/1 -> SetPointGuiHandler/2(target_torque)
  omega/1 -> SetPointGuiHandler/5(omega)
  control_reset_switch/1 -> SetPointGuiHandler/6(control_reset_switch)
  SetPointGuiHandler/4(control_strategy) -> control strategy/1
  SetPointGuiHandler/3(target_torque_out) -> target_torque_out/1
  SetPointGuiHandler/1(target_postion_out) -> target_position_out/1
  SetPointGuiHandler/2(target_velocity_out) -> target_velocity_out/1

== system SomanetTuning/Slider ==

== system SomanetTuning/Slider1 ==

== system SomanetTuning/Slider10 ==

== system SomanetTuning/Slider11 ==

== system SomanetTuning/Slider12 ==

== system SomanetTuning/Slider13 ==

== system SomanetTuning/Slider2 ==

== system SomanetTuning/Slider3 ==

== system SomanetTuning/Slider4 ==

== system SomanetTuning/Slider5 ==

== system SomanetTuning/Slider6 ==

== system SomanetTuning/Slider7 ==

== system SomanetTuning/Slider8 ==

== system SomanetTuning/Slider9 ==

== system SomanetTuning/Toggle Switch ==

== system SomanetTuning/Toggle Switch1 ==

== system SomanetTuning/Toggle Switch2 ==

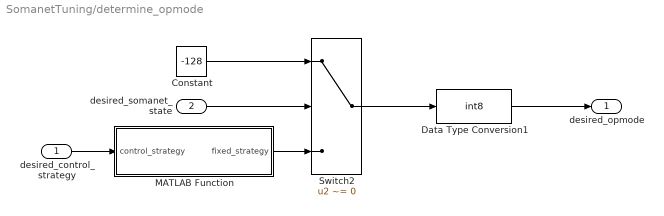
== system SomanetTuning/determine_opmode ==
  desired_control_strategy : Inport
  desired_somanet_state : Inport  Port=2
  Constant : Constant  Value=-128
  Data Type Conversion1 : DataTypeConversion  OutDataTypeStr=int8
  MATLAB Function : MATLAB Function  TreatAsAtomicUnit=on
  Switch2 : Switch  Criteria=u2 ~= 0
  desired_opmode : Outport
  wires:
  Constant/1 -> Switch2/1
  Switch2/1 -> Data Type Conversion1/1
  desired_somanet_state/1 -> Switch2/2
  desired_control_strategy/1 -> MATLAB Function/1(control_strategy)
  Data Type Conversion1/1 -> desired_opmode/1
  MATLAB Function/1(fixed_strategy) -> Switch2/3
